simulink model "SimulinkModel_ReadEncoderData_SendMotorCommands"  (R2018a)
settings: Solver=VariableStepAuto  StartTime=0.0  StopTime=inf  RelTol=1e-3
libraries: robotlib x6, aerolibanimutils x1
settings Model: Creator=uvsgta  LastModifiedBy=askar

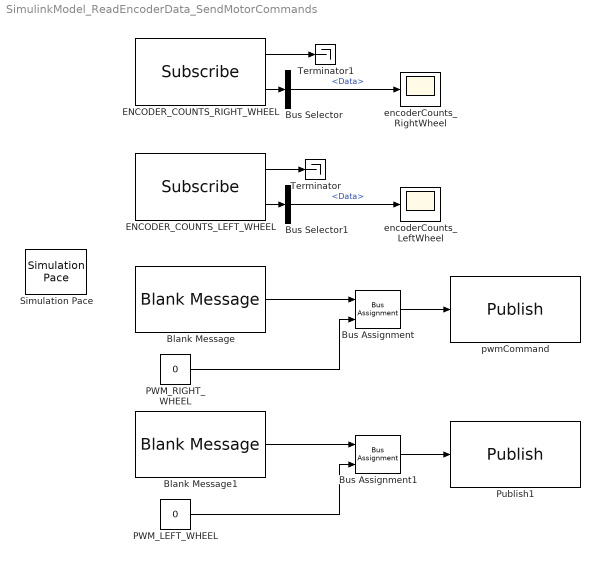
== system SimulinkModel_ReadEncoderData_SendMotorCommands ==
  Blank Message : robotlib/Blank Message  SourceLibraryInfo=This block requires Robotics System Toolbox  messageType=std_msgs/Int16  SampleTime=inf
      settings: SourceProductBaseCode=RO
  Blank Message1 : robotlib/Blank Message  SourceLibraryInfo=This block requires Robotics System Toolbox  messageType=std_msgs/Int16  SampleTime=inf
      settings: SourceProductBaseCode=RO
  Bus Assignment : BusAssignment  AssignedSignals=Data
  Bus Assignment1 : BusAssignment  AssignedSignals=Data
  Bus Selector : BusSelector  OutputSignals=Data
  Bus Selector1 : BusSelector  OutputSignals=Data
  ENCODER_COUNTS_LEFT_WHEEL : robotlib/Subscribe  SourceLibraryInfo=This block requires Robotics System Toolbox  topicSource=Select from ROS network  topic=/enco_L  messageType=std_msgs/Int16  sampleTime=-1  messageQueueLength=1
      settings: SourceProductBaseCode=RO
  ENCODER_COUNTS_RIGHT_WHEEL : robotlib/Subscribe  SourceLibraryInfo=This block requires Robotics System Toolbox  topicSource=Select from ROS network  topic=/enco_R  messageType=std_msgs/Int16  sampleTime=-1  messageQueueLength=1
      settings: SourceProductBaseCode=RO
  PWM_LEFT_WHEEL : Constant  Value=0  OutDataTypeStr=int16
  PWM_RIGHT_WHEEL : Constant  Value=0  OutDataTypeStr=int16
  Publish1 : robotlib/Publish  SourceLibraryInfo=This block requires Robotics System Toolbox  topicSource=Select from ROS network  topic=/pwm_cmd_l  messageType=std_msgs/Int16  messageQueueLength=1
      settings: SourceProductBaseCode=RO
  Simulation Pace : aerolibanimutils/Simulation Pace  SimulationPace=1  SleepMode=MATLAB Thread  OutputPaceError=off  SampleTime=1/30
  Terminator : Terminator
  Terminator1 : Terminator
  encoderCounts_LeftWheel : Scope
  encoderCounts_RightWheel : Scope
  pwmCommand : robotlib/Publish  SourceLibraryInfo=This block requires Robotics System Toolbox  topicSource=Select from ROS network  topic=/pwm_cmd_r  messageType=std_msgs/Int16  messageQueueLength=1
      settings: SourceProductBaseCode=RO
  wires:
  ENCODER_COUNTS_RIGHT_WHEEL/2 -> Bus Selector/1
  Bus Selector/1 -> encoderCounts_RightWheel/1  "<Data>"
  Bus Selector1/1 -> encoderCounts_LeftWheel/1  "<Data>"
  ENCODER_COUNTS_LEFT_WHEEL/2 -> Bus Selector1/1
  ENCODER_COUNTS_LEFT_WHEEL/1 -> Terminator/1
  ENCODER_COUNTS_RIGHT_WHEEL/1 -> Terminator1/1
  Blank Message/1 -> Bus Assignment/1
  Bus Assignment/1 -> pwmCommand/1
  PWM_RIGHT_WHEEL/1 -> Bus Assignment/2
  PWM_LEFT_WHEEL/1 -> Bus Assignment1/2
  Bus Assignment1/1 -> Publish1/1
  Blank Message1/1 -> Bus Assignment1/1
